simulink model "gm_ObjectTrackerHDL"  (R2024a)
settings: Solver=VariableStepAuto  StartTime=0.0  StopTime=5.5  RelTol=1e-3  EnableMultiTasking=on
PreLoadFcn:
  | % Blank input
  | img = zeros(480,640);
  | 
  | % Initialize ROI and its center
  | ROI = [175 270 127 127];
  | center = [ROI(2)+(ROI(4)+1)/2 ROI(1)+(ROI(3)+1)/2];
  | 
  | % Template Size
  | templateSize = 128;
  | tSize = templateSize;
  | 
  | % Learning rate
  | eta = 0.075;
  | 
  | % Number of training images
  | trainCount = 2;
  | 
  | % Gaussian Variance
  | sig = 2;
  | 
  | % Generate a Gaussian centered on the first frame
  | iSize = size(img);
  | [x,y] = ndgrid(1:iSize(1), 1:iSize(2));
  | gauss = exp(-((x-center(1)).^2 + (y-center(2)).^2)./(2*sig));
  | gauss = mat2gray(gauss);
  | 
  | % Generate the first template
  | img = imcrop(img, ROI);
  | gauss = imcrop(gauss, ROI);
  | 
  | % Generate the preprocess windowing function
  | [w1,w2] = meshgrid(window(@hann,tSize),window(@hann,tSize));
  | win = w1.*w2;
  | 
  | % Blank initial coefficients
  | G = zeros(tSize,tSize);
  | Ai = zeros(tSize,tSize);
  | Bi = zeros(tSize,tSize);
  | Hi = zeros(tSize,tSize);
  | 
  | numRows = tSize;
  | numCols = tSize;
InitFcn:
  | % Read the first frame
  | vidFReader = VideoReader(get_param('ObjectTrackerHDL/Input','inputFilename'));
  | img = read(vidFReader,1);
  | if (size(img,3) == 3)
  |     img = rgb2gray(img);
  | end
  | img = double(img);
  | 
  | % Initialize Object Center
  | objectCenter = str2num(get_param('ObjectTrackerHDL/ObjectTrackerHDL','objectCenter'));
  | 
  | % Template Size
  | templateSize = str2num(get_param('ObjectTrackerHDL/ObjectTrackerHDL','templateSize'));
  | originROI = objectCenter-templateSize/2;
  | tSize = templateSize;
  | 
  | % Initialize ROI and its center
  | ROI = [originROI tSize-1 tSize-1];
  | center = [ROI(2)+(ROI(4)+1)/2 ROI(1)+(ROI(3)+1)/2];
  | 
  | % Learning rate
  | eta = 0.075;
  | 
  | % Number of training images
  | trainCount = 128;
  | 
  | % Gaussian Variance
  | sig = 2;
  | 
  | % Generate a Gaussian centered on the first frame
  | iSize = size(img);
  | [x,y] = ndgrid(1:iSize(1), 1:iSize(2));
  | gauss = exp(-((x-center(1)).^2 + (y-center(2)).^2)./(2*sig));
  | gauss = mat2gray(gauss);
  | 
  | % Generate the first template
  | img = imcrop(img, ROI);
  | gauss = imcrop(gauss, ROI);
  | 
  | % Generate the preprocess windowing function
  | [w1,w2] = meshgrid(window(@hann,tSize),window(@hann,tSize));
  | win = w1.*w2;
  | 
  | % Preprocessing the first template
  | hgamma = vision.GammaCorrector(2.0,'Correction','De-gamma');
  | img = hgamma(uint8(img));
  | img = double(img);
  | mean1 = mean(img(:));
  | std1 = std(img(:));
  | img = (img-mean1)/std1;
  | fii = img.*win;
  | 
  | % Convert to frequency domain and calculate initial coefficients
  | G = fft2(gauss);
  | Ai = (G.*conj(fft2(fii)));
  | Bi = real((fft2(fii).*conj(fft2(fii))));
  | 
  | rng('default');
  | % Initial training procedure
  | for i = 1:trainCount
  | ... (+19 lines)
model workspace (MAT data in the model file):
  mwTaskManagerKernelLatency = 0
undefined symbols (not defined in the file or in its folder): a, b, c, Rec, SDTV
libraries: hdlsllib x61, simulink x17, visionhdlutilities x8, visionstatistics x6, dsphdlxfrm2 x6, visionconversions x3, visiontransforms x3, visionhdlio x2, visionhdlconversions x2, visionhdlstatistics x2, visionsinks x1, dspvision x1
(part 2 of 3)

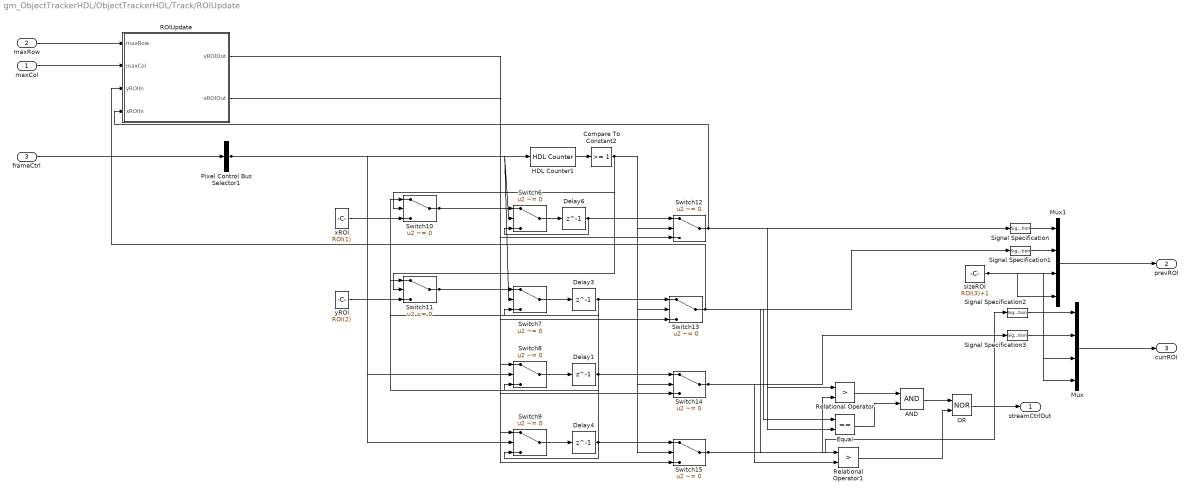
== system gm_ObjectTrackerHDL/ObjectTrackerHDL/Track/ROIUpdate ==
  maxCol : Inport  OutDataTypeStr=uint16  PortDimensions=1  SampleTime=7.94444444444444e-08
  maxRow : Inport  Port=2  OutDataTypeStr=uint16  PortDimensions=1  SampleTime=7.94444444444444e-08
  frameCtrl : Inport  Port=3
  AND : Logic  AllPortsSameDT=off  OutDataTypeStr=boolean
  Compare To Constant2 : simulink/Logic and Bit Operations/Compare To Constant  relop=>=  const=1  OutDataTypeStr=boolean
  Delay{1,3..4,6} (4 alike) : Delay  DelayLength=1
  Equal : RelationalOperator  Operator===  OutDataTypeStr=boolean  RndMeth=Simplest  InputSameDT=off
  HDL Counter1 : hdlsllib/Sources/HDL Counter  CountType=Count limited  CountInit=0  CountStep=1  CountMax=4095  CountFromType=Initial value  CountFrom=0  CountResetPort=off  CountLoadPort=off  CountEnbPort=on  CountDirPort=off  CountHitOutputPort=off  CountDataType=Unsigned  CountWordLen=12  CountFracLen=0  CountSampTime=1
  Mux : Mux
  Mux1 : Mux
  OR : Logic  Operator=NOR  AllPortsSameDT=off  OutDataTypeStr=boolean
  Pixel Control Bus Selector1 : BusSelector  OutputSignals=vEnd
  ROIUpdate : Subsystem
  Relational Operator : RelationalOperator  Operator=>  OutDataTypeStr=boolean  RndMeth=Simplest  InputSameDT=off
  Relational Operator1 : RelationalOperator  Operator=>  OutDataTypeStr=boolean  RndMeth=Simplest  InputSameDT=off
  Signal Specification{,1..3} (4 alike) : SignalSpecification  OutDataTypeStr=uint16  Dimensions=1
  Switch{6..7,10..15} (8 alike) : Switch  Criteria=u2 ~= 0  OutDataTypeStr=uint16  SaturateOnIntegerOverflow=off  InputSameDT=off
  Switch8 : Switch  Criteria=u2 ~= 0  OutDataTypeStr=fixdt(1, 17, 0)  SaturateOnIntegerOverflow=off  InputSameDT=off
  Switch9 : Switch  Criteria=u2 ~= 0  OutDataTypeStr=fixdt(1, 17, 0)  SaturateOnIntegerOverflow=off  InputSameDT=off
  sizeROI : Constant  Value=ROI(3)+1  OutDataTypeStr=uint16  SampleTime=-1
  xROI : Constant  Value=ROI(1)  OutDataTypeStr=uint16  SampleTime=-1
  yROI : Constant  Value=ROI(2)  OutDataTypeStr=uint16  SampleTime=-1
  streamCtrlOut : Outport  SampleTime=7.94444444444444e-08
  prevROI : Outport  Port=2  SampleTime=7.94444444444444e-08
  currROI : Outport  Port=3  SampleTime=7.94444444444444e-08
  wires:
  frameCtrl/1 -> Pixel Control Bus Selector1/1
  AND/1 -> OR/1
  Compare To Constant2/1 -> Switch15/2, Switch14/2, Switch13/2, Switch12/2, Switch11/2, Switch10/2
  Delay1/1 -> Switch14/1, Switch8/3, Switch11/1
  Delay4/1 -> Switch15/1, Switch9/3, Switch10/1
  Equal/1 -> AND/2
  HDL Counter1/1 -> Compare To Constant2/1
  Mux/1 -> currROI/1
  Mux1/1 -> prevROI/1
  OR/1 -> streamCtrlOut/1
  Pixel Control Bus Selector1/1 -> Switch9/2, Switch8/2, Switch7/2, Switch6/2, HDL Counter1/1
  Relational Operator/1 -> AND/1
  Relational Operator1/1 -> OR/2
  Signal Specification/1 -> Mux1/1
  Signal Specification1/1 -> Mux1/2
  Signal Specification2/1 -> Mux/1
  Signal Specification3/1 -> Mux/2
  Switch10/1 -> Switch15/3, Switch6/1, Switch12/3
  Switch11/1 -> Switch14/3, Switch7/1, Switch13/3
  Switch12/1 -> Relational Operator/1, Signal Specification/1, ROIUpdate/4(xROIIn)
  Switch13/1 -> Relational Operator1/1, Equal/1, Signal Specification1/1, ROIUpdate/3(yROIIn)
  Switch14/1 -> Relational Operator1/2, Equal/2, Signal Specification3/1
  Switch15/1 -> Relational Operator/2, Signal Specification2/1
  sizeROI/1 -> Mux1/4, Mux1/3, Mux/4, Mux/3
  Delay6/1 -> Switch12/1, Switch6/3
  Delay3/1 -> Switch13/1, Switch7/3
  xROI/1 -> Switch10/3
  yROI/1 -> Switch11/3
  maxRow/1 -> ROIUpdate/1(maxRow)
  maxCol/1 -> ROIUpdate/2(maxCol)
  Switch6/1 -> Delay6/1
  Switch8/1 -> Delay1/1
  Switch7/1 -> Delay3/1
  Switch9/1 -> Delay4/1
  ROIUpdate/1(yROIOut) -> Switch8/1
  ROIUpdate/2(xROIOut) -> Switch9/1

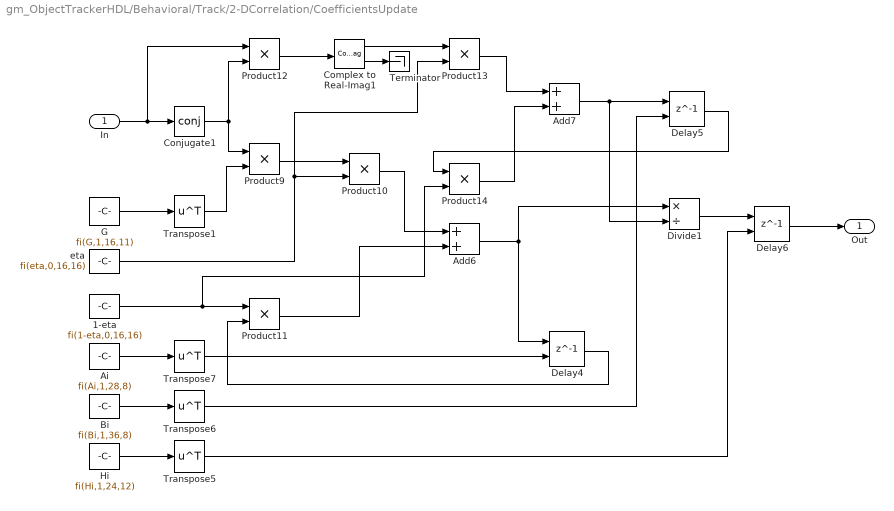
== system gm_ObjectTrackerHDL/Behavioral/Track/2-DCorrelation/CoefficientsUpdate ==
  In : Inport
  1-eta : Constant  Value=fi(1-eta,0,16,16)  OutDataTypeStr=fixdt(0,16,16)  SampleTime=-1
  Add6 : Sum  OutDataTypeStr=fixdt(1,28,8)
  Add7 : Sum  OutDataTypeStr=fixdt(1,36,8)
  Ai : Constant  Value=fi(Ai,1,28,8)  OutDataTypeStr=fixdt(1,28,8)  SampleTime=-1
  Bi : Constant  Value=fi(Bi,1,36,8)  OutDataTypeStr=fixdt(1,36,8)  SampleTime=-1
  Complex to Real-Imag1 : ComplexToRealImag
  Conjugate1 : Math  Operator=conj  SignedPower=on  RndMeth=Zero
  Delay4 : Delay  DelayLength=1  InitialConditionSource=Input port  InitialCondition=Ai
      settings: InputPortMap=u0,p4
  Delay5 : Delay  DelayLength=1  InitialConditionSource=Input port  InitialCondition=Bi
      settings: InputPortMap=u0,p4
  Delay6 : Delay  DelayLength=1  InitialConditionSource=Input port  InitialCondition=Hi
      settings: InputPortMap=u0,p4
  Divide1 : Product  Inputs=*/  OutDataTypeStr=fixdt(1,24,12)  RndMeth=Simplest  SaturateOnIntegerOverflow=on
  G : Constant  Value=fi(G,1,16,11)  VectorParams1D=off  SampleTime=-1
  Hi : Constant  Value=fi(Hi,1,24,12)  OutDataTypeStr=fixdt(1,24,12)  SampleTime=-1
  Product10 : Product  OutDataTypeStr=fixdt(1,24,12)
  Product11 : Product  OutDataTypeStr=fixdt(1,28,8)
  Product12 : Product  OutDataTypeStr=fixdt(1,32,8)
  Product13 : Product  OutDataTypeStr=fixdt(1,32,12)
  Product14 : Product  OutDataTypeStr=fixdt(1,36,8)
  Product9 : Product  OutDataTypeStr=fixdt(1,24,8)
  Terminator : Terminator
  Transpose{1,5..7} (4 alike) : Math  Operator=transpose
  eta : Constant  Value=fi(eta,0,16,16)  SampleTime=-1
  Out : Outport
  wires:
  Transpose1/1 -> Product9/2
  Delay4/1 -> Product11/2
  Transpose7/1 -> Delay4/2
  Transpose5/1 -> Delay6/2
  Product12/1 -> Complex to Real-Imag1/1
  Bi/1 -> Transpose6/1
  Delay6/1 -> Out/1
  Complex to Real-Imag1/1 -> Product13/1
  Complex to Real-Imag1/2 -> Terminator/1
  G/1 -> Transpose1/1
  Product13/1 -> Add7/1
  Delay5/1 -> Product14/1
  Product10/1 -> Add6/1
  Hi/1 -> Transpose5/1
  Add7/1 -> Divide1/2, Delay5/1
  Transpose6/1 -> Delay5/2
  1-eta/1 -> Product14/2, Product11/1
  Product11/1 -> Add6/2
  Conjugate1/1 -> Product9/1, Product12/2
  Product9/1 -> Product10/1
  In/1 -> Conjugate1/1, Product12/1
  eta/1 -> Product10/2, Product13/2
  Divide1/1 -> Delay6/1
  Add6/1 -> Divide1/1, Delay4/1
  Ai/1 -> Transpose7/1
  Product14/1 -> Add7/2

== system gm_ObjectTrackerHDL/Behavioral/Track/ROIUpdate/CurrValidROI ==
  ROIIn : Inport
  Constant : Constant  Value=iSize(1)-tSize  OutDataTypeStr=uint16  SampleTime=-1
  Constant1 : Constant  Value=iSize(2)-tSize  OutDataTypeStr=uint16  SampleTime=-1
  Demux : Demux
  Mux1 : Mux
  Relational Operator : RelationalOperator  Operator=<  OutDataTypeStr=boolean  RndMeth=Simplest  InputSameDT=off
  Relational Operator1 : RelationalOperator  Operator=<  OutDataTypeStr=boolean  RndMeth=Simplest  InputSameDT=off
  Switch : Switch  Criteria=u2 ~= 0  SaturateOnIntegerOverflow=off  InputSameDT=off
  Switch1 : Switch  Criteria=u2 ~= 0  SaturateOnIntegerOverflow=off  InputSameDT=off
  ROIOut : Outport
  wires:
  Switch1/1 -> Mux1/2
  Relational Operator1/1 -> Switch1/2
  Switch/1 -> Mux1/1
  Relational Operator/1 -> Switch/2
  Demux/4 -> Mux1/4
  Demux/3 -> Mux1/3
  Constant/1 -> Relational Operator1/2, Switch1/3
  Demux/2 -> Switch1/1, Relational Operator1/1
  Constant1/1 -> Relational Operator/2, Switch/3
  Demux/1 -> Relational Operator/1, Switch/1
  ROIIn/1 -> Demux/1
  Mux1/1 -> ROIOut/1

== system gm_ObjectTrackerHDL/Behavioral/Track/ROIUpdate/PrevValidROI ==
  ROIIn : Inport
  Constant : Constant  Value=iSize(1)-tSize  OutDataTypeStr=uint16  SampleTime=-1
  Constant1 : Constant  Value=iSize(2)-tSize  OutDataTypeStr=uint16  SampleTime=-1
  Demux : Demux
  Mux1 : Mux
  Relational Operator : RelationalOperator  Operator=<  OutDataTypeStr=boolean  RndMeth=Simplest  InputSameDT=off
  Relational Operator1 : RelationalOperator  Operator=<  OutDataTypeStr=boolean  RndMeth=Simplest  InputSameDT=off
  Switch : Switch  Criteria=u2 ~= 0  SaturateOnIntegerOverflow=off  InputSameDT=off
  Switch1 : Switch  Criteria=u2 ~= 0  SaturateOnIntegerOverflow=off  InputSameDT=off
  ROIOut : Outport
  wires:
  Switch1/1 -> Mux1/2
  Relational Operator1/1 -> Switch1/2
  Switch/1 -> Mux1/1
  Relational Operator/1 -> Switch/2
  Demux/4 -> Mux1/4
  Demux/3 -> Mux1/3
  Constant/1 -> Relational Operator1/2, Switch1/3
  Demux/2 -> Switch1/1, Relational Operator1/1
  Constant1/1 -> Relational Operator/2, Switch/3
  Demux/1 -> Relational Operator/1, Switch/1
  ROIIn/1 -> Demux/1
  Mux1/1 -> ROIOut/1

== system gm_ObjectTrackerHDL/ObjectTrackerHDL/Overlay/VideoOverlay/Divide ==
  In1 : Inport
  In2 : Inport  Port=2
  Divide : Product  Inputs=*/  OutDataTypeStr=fixdt(1, 18, 0)  RndMeth=Zero  SaturateOnIntegerOverflow=on
  Divide_pd1 : Delay  DelayLength=22
  Out1 : Outport
  wires:
  In1/1 -> Divide/1
  In2/1 -> Divide/2
  Divide/1 -> Divide_pd1/1
  Divide_pd1/1 -> Out1/1

== system gm_ObjectTrackerHDL/ObjectTrackerHDL/Overlay/VideoOverlay/MATLAB Function ==
  position : Inport  OutDataTypeStr=uint16  PortDimensions=[1 4]  SampleTime=7.94444444444444e-08
  rowCount : Inport  Port=2  OutDataTypeStr=int32  PortDimensions=1  SampleTime=7.94444444444444e-08
  colCount : Inport  Port=3  OutDataTypeStr=int32  PortDimensions=1  SampleTime=7.94444444444444e-08
  colorValue : Inport  Port=4  OutDataTypeStr=uint8  PortDimensions=[1 3]  SampleTime=7.94444444444444e-08
  lineWidth : Inport  Port=5  OutDataTypeStr=uint8  PortDimensions=1  SampleTime=7.94444444444444e-08
  MATLAB Function : MATLAB Function  TreatAsAtomicUnit=on
  Color : Outport  SampleTime=7.94444444444444e-08  VectorParamsAs1DForOutWhenUnconnected=off
  AddShape : Outport  Port=2  SampleTime=7.94444444444444e-08
  wires:
  position/1 -> MATLAB Function/1(position)
  rowCount/1 -> MATLAB Function/2(rowCount)
  colCount/1 -> MATLAB Function/3(colCount)
  colorValue/1 -> MATLAB Function/4(colorValue)
  lineWidth/1 -> MATLAB Function/5(lineWidth)
  MATLAB Function/1(Color) -> Color/1
  MATLAB Function/2(AddShape) -> AddShape/1

== system gm_ObjectTrackerHDL/ObjectTrackerHDL/Preprocess/CurrPreprocess/Divide1 ==
  In1 : Inport
  In2 : Inport  Port=2
  Divide1 : Product  Inputs=*/  OutDataTypeStr=fixdt(1,16,12)  RndMeth=Zero  SaturateOnIntegerOverflow=on
  Divide1_pd1 : Delay  DelayLength=34
  Out1 : Outport
  wires:
  In1/1 -> Divide1/1
  In2/1 -> Divide1/2
  Divide1/1 -> Divide1_pd1/1
  Divide1_pd1/1 -> Out1/1

== system gm_ObjectTrackerHDL/ObjectTrackerHDL/Preprocess/CurrPreprocess/Multiply_ShiftAdd_inst ==
  In1 : Inport
  In2 : Inport  Port=2
  Multiply_ShiftAdd_inst : Product  OutDataTypeStr=fixdt(1, 32, 28)
  Multiply_ShiftAdd_inst_pd1 : Delay  DelayLength=4
  Out1 : Outport
  wires:
  In1/1 -> Multiply_ShiftAdd_inst/1
  In2/1 -> Multiply_ShiftAdd_inst/2
  Multiply_ShiftAdd_inst_pd1/1 -> Out1/1
  Multiply_ShiftAdd_inst/1 -> Multiply_ShiftAdd_inst_pd1/1

== system gm_ObjectTrackerHDL/ObjectTrackerHDL/Preprocess/PrevPreprocess/Divide2 ==
  In1 : Inport
  In2 : Inport  Port=2
  Divide2 : Product  Inputs=*/  OutDataTypeStr=fixdt(1,16,12)  RndMeth=Zero  SaturateOnIntegerOverflow=on
  Divide2_pd1 : Delay  DelayLength=34
  Out1 : Outport
  wires:
  In1/1 -> Divide2/1
  In2/1 -> Divide2/2
  Divide2/1 -> Divide2_pd1/1
  Divide2_pd1/1 -> Out1/1

== system gm_ObjectTrackerHDL/ObjectTrackerHDL/Preprocess/PrevPreprocess/Multiply_ShiftAdd_inst ==
  In1 : Inport
  In2 : Inport  Port=2
  Multiply_ShiftAdd_inst : Product  OutDataTypeStr=fixdt(1, 32, 28)
  Multiply_ShiftAdd_inst_pd1 : Delay  DelayLength=4
  Out1 : Outport
  wires:
  In1/1 -> Multiply_ShiftAdd_inst/1
  In2/1 -> Multiply_ShiftAdd_inst/2
  Multiply_ShiftAdd_inst_pd1/1 -> Out1/1
  Multiply_ShiftAdd_inst/1 -> Multiply_ShiftAdd_inst_pd1/1

== system gm_ObjectTrackerHDL/ObjectTrackerHDL/Track/2-DCorrelation/2-DIFFT ==
  pixelIn : Inport  OutDataTypeStr=fixdt(1, 24, 16)  PortDimensions=1  SampleTime=7.94444444444444e-08
      settings: SignalType=complex
  ctrlIn : Inport  Port=2
  " " : DataTypeConversion  OutDataTypeStr=fixdt(1,24,16)  SaturateOnIntegerOverflow=off  RndMeth=Floor
  Bit Concat1 : hdlsllib/Logic and Bit Operations/Bit Concat  numInputs=2
  Bit Slice4 : hdlsllib/Logic and Bit Operations/Bit Slice  lidx=31  ridx=0
  Bit Slice5 : hdlsllib/Logic and Bit Operations/Bit Slice  lidx=63  ridx=32
  ColumnIFFT : dsphdlxfrm2/IFFT  Architecture=Streaming Radix 2^2  FFTLengthSource=Property  FFTLength=tSize  FFTLengthMax=1024  ComplexMultiplication=Use 4 multipliers and 2 adders  BitReversedOutput=off  BitReversedInput=off  Normalize=on  SimulateUsing=Code generation  RoundingMethod=Floor  ResetInputPort=off  StartOutputPort=off  EndOutputPort=off
  Complex to Real-Imag : ComplexToRealImag
  Complex to Real-Imag1 : ComplexToRealImag
  Complex to Real-Imag_term1 : Terminator
  CornerTurnMemory : Subsystem
  Data Type Conversion10 : DataTypeConversion  OutDataTypeStr=fixdt(1,24,16)  SaturateOnIntegerOverflow=off  RndMeth=Floor
  Data Type Conversion12 : DataTypeConversion  OutDataTypeStr=fixdt(1,24,16)  SaturateOnIntegerOverflow=off  RndMeth=Floor
  Data Type Conversion8 : DataTypeConversion  OutDataTypeStr=fixdt(0,32,0)  ConvertRealWorld=Stored Integer (SI)  SaturateOnIntegerOverflow=off  RndMeth=Floor
  Data Type Conversion9 : DataTypeConversion  OutDataTypeStr=fixdt(1,24,16)  ConvertRealWorld=Stored Integer (SI)  SaturateOnIntegerOverflow=off  RndMeth=Floor
  Pixel Control Bus Selector1 : BusSelector  OutputSignals=valid
  Real-Imag to Complex1 : RealImagToComplex
  RowIFFT : dsphdlxfrm2/IFFT  Architecture=Streaming Radix 2^2  FFTLengthSource=Property  FFTLength=tSize  FFTLengthMax=1024  ComplexMultiplication=Use 4 multipliers and 2 adders  BitReversedOutput=off  BitReversedInput=off  Normalize=on  SimulateUsing=Code generation  RoundingMethod=Floor  ResetInputPort=off  StartOutputPort=off  EndOutputPort=off
  pixelBusGenerator : Subsystem  mask{hEnd=double(127), vEnd=double(16383)}
      mask prompts: hEnd "hEnd Count"; vEnd "vEnd Count"
  pixelOut : Outport  SampleTime=7.94444444444444e-08
  ctrlOut : Outport  Port=2
  wires:
  pixelIn/1 -> Data Type Conversion10/1
  ctrlIn/1 -> Pixel Control Bus Selector1/1
  " "/1 -> Complex to Real-Imag/1
  Bit Concat1/1 -> CornerTurnMemory/1(dataIn)
  Bit Slice4/1 -> Real-Imag to Complex1/2
  Bit Slice5/1 -> Real-Imag to Complex1/1
  ColumnIFFT/1 -> " "/1
  ColumnIFFT/2 -> pixelBusGenerator/1(validIn)
  Complex to Real-Imag/1 -> pixelOut/1
  Complex to Real-Imag/2 -> Complex to Real-Imag_term1/1
  Complex to Real-Imag1/1 -> Bit Concat1/1
  Complex to Real-Imag1/2 -> Bit Concat1/2
  CornerTurnMemory/1(dataOut) -> Bit Slice5/1, Bit Slice4/1
  CornerTurnMemory/2(validOut) -> ColumnIFFT/2
  Data Type Conversion10/1 -> RowIFFT/1
  Data Type Conversion12/1 -> Data Type Conversion8/1
  Data Type Conversion8/1 -> Complex to Real-Imag1/1
  Data Type Conversion9/1 -> ColumnIFFT/1
  Pixel Control Bus Selector1/1 -> RowIFFT/2
  Real-Imag to Complex1/1 -> Data Type Conversion9/1
  RowIFFT/1 -> Data Type Conversion12/1
  RowIFFT/2 -> CornerTurnMemory/2(validIn)
  pixelBusGenerator/1(busOut) -> ctrlOut/1

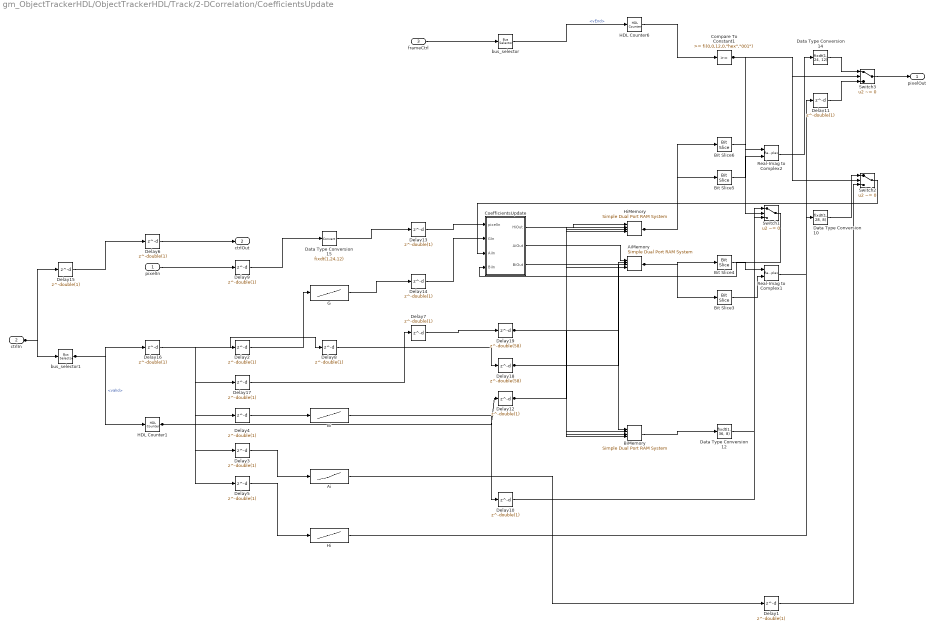
== system gm_ObjectTrackerHDL/ObjectTrackerHDL/Track/2-DCorrelation/CoefficientsUpdate ==
  pixelIn : Inport  OutDataTypeStr=fixdt(1, 24, 12)  PortDimensions=1  SampleTime=7.94444444444444e-08
      settings: SignalType=complex
  ctrlIn : Inport  Port=2
  frameCtrl : Inport  Port=3
  Ai : Lookup_n-D  NumberOfTableDimensions=1  LookupTableObject=''  BreakpointsForDimension1=[0:tSize * tSize - 1]  BreakpointsForDimension1FirstPoint=10  BreakpointsForDimension2FirstPoint=10  BreakpointsForDimension1Spacing=12  BreakpointsForDimension2Spacing=12  IndexSearchMethod=Evenly spaced points  Table=fi(Ai(:),1,28,8)  InterpMethod=Flat  InternalRulePriority=Speed  OutDataTypeStr=fixdt(1,28,8)  RndMeth=Simplest
  AiMemory : hdlsllib/HDL RAMs/Simple Dual Port RAM System  RAMType=Simple dual port  AsyncRead=off  WriteOutputValue=New data  RAMInitialValue=0  allowBusInputs=off  WritesHaveOutput=on  NumReads=0  NumWrites=1  SimulateUsing=Code generation
  Bi : Lookup_n-D  NumberOfTableDimensions=1  LookupTableObject=''  BreakpointsForDimension1=[0:tSize * tSize - 1]  BreakpointsForDimension1FirstPoint=10  BreakpointsForDimension2FirstPoint=10  BreakpointsForDimension1Spacing=12  BreakpointsForDimension2Spacing=12  IndexSearchMethod=Evenly spaced points  Table=fi(Bi(:),1,36,8)  InterpMethod=Flat  InternalRulePriority=Speed  OutDataTypeStr=fixdt(1,36,8)  RndMeth=Simplest
  BiMemory : hdlsllib/HDL RAMs/Simple Dual Port RAM System  RAMType=Simple dual port  AsyncRead=off  WriteOutputValue=New data  RAMInitialValue=0  allowBusInputs=off  WritesHaveOutput=on  NumReads=0  NumWrites=1  SimulateUsing=Code generation
  Bit Slice3 : hdlsllib/Logic and Bit Operations/Bit Slice  lidx=double(31)  ridx=double(0)
  Bit Slice4 : hdlsllib/Logic and Bit Operations/Bit Slice  lidx=double(63)  ridx=double(32)
  Bit Slice5 : hdlsllib/Logic and Bit Operations/Bit Slice  lidx=double(31)  ridx=double(0)
  Bit Slice6 : hdlsllib/Logic and Bit Operations/Bit Slice  lidx=double(63)  ridx=double(32)
  CoefficientsUpdate : Subsystem
  Compare To Constant1 : simulink/Logic and Bit Operations/Compare To Constant  relop=>=  const="fi(0,0,12,0,\"hex\",\"001\")"  OutDataTypeStr=boolean
  Data Type Conversion10 : DataTypeConversion  OutDataTypeStr=fixdt(1, 28, 8)  ConvertRealWorld=Stored Integer (SI)  SampleTime=7.94444444444444e-08  SaturateOnIntegerOverflow=off  RndMeth=Floor
  Data Type Conversion12 : DataTypeConversion  OutDataTypeStr=fixdt(1, 36, 8)  ConvertRealWorld=Stored Integer (SI)  SampleTime=7.94444444444444e-08  SaturateOnIntegerOverflow=off  RndMeth=Floor
  Data Type Conversion14 : DataTypeConversion  OutDataTypeStr=fixdt(1, 24, 12)  ConvertRealWorld=Stored Integer (SI)  SampleTime=7.94444444444444e-08  SaturateOnIntegerOverflow=off  RndMeth=Floor
  Data Type Conversion15 : DataTypeConversion  OutDataTypeStr=fixdt(1,24,12)
  Delay{1..5,7..14,16..17} (15 alike) : Delay  DelayLength=double(1)  InitialCondition=0  SampleTime=7.94444444444444e-08
  Delay15 : Delay  DelayLength=double(1)  SampleTime=7.94444444444444e-08
  Delay18 : Delay  DelayLength=double(58)  InitialCondition=0  SampleTime=7.94444444444444e-08
  Delay19 : Delay  DelayLength=double(58)  InitialCondition=0  SampleTime=7.94444444444444e-08
  Delay6 : Delay  DelayLength=double(1)  SampleTime=7.94444444444444e-08
  G : Lookup_n-D  NumberOfTableDimensions=1  LookupTableObject=''  BreakpointsForDimension1=[0:tSize * tSize - 1]  BreakpointsForDimension1FirstPoint=10  BreakpointsForDimension2FirstPoint=10  BreakpointsForDimension1Spacing=12  BreakpointsForDimension2Spacing=12  IndexSearchMethod=Evenly spaced points  Table=fi(G(:),1,16,11)  InterpMethod=Flat  InternalRulePriority=Speed  OutDataTypeStr=fixdt(1,16,11)  RndMeth=Simplest
  HDL Counter1 : hdlsllib/Sources/HDL Counter  CountType=Count limited  CountInit=0  CountStep=1  CountMax=tSize * tSize - 1  CountFromType=Initial value  CountFrom=0  CountResetPort=off  CountLoadPort=off  CountEnbPort=on  CountDirPort=off  CountHitOutputPort=off  CountDataType=Unsigned  CountWordLen=ceil(log2(tSize * tSize - 1))  CountFracLen=0  CountSampTime=1
  HDL Counter6 : hdlsllib/Sources/HDL Counter  CountType=Count limited  CountInit=0  CountStep=1  CountMax=4095  CountFromType=Initial value  CountFrom=0  CountResetPort=off  CountLoadPort=off  CountEnbPort=on  CountDirPort=off  CountHitOutputPort=off  CountDataType=Unsigned  CountWordLen=12  CountFracLen=0  CountSampTime=1
  Hi : Lookup_n-D  NumberOfTableDimensions=1  LookupTableObject=''  BreakpointsForDimension1=[0:tSize * tSize - 1]  BreakpointsForDimension1FirstPoint=10  BreakpointsForDimension2FirstPoint=10  BreakpointsForDimension1Spacing=12  BreakpointsForDimension2Spacing=12  IndexSearchMethod=Evenly spaced points  Table=fi(Hi(:),1,24,12)  InterpMethod=Flat  InternalRulePriority=Speed  OutDataTypeStr=fixdt(1,24,12)  RndMeth=Simplest
  HiMemory : hdlsllib/HDL RAMs/Simple Dual Port RAM System  RAMType=Simple dual port  AsyncRead=off  WriteOutputValue=New data  RAMInitialValue=0  allowBusInputs=off  WritesHaveOutput=on  NumReads=0  NumWrites=1  SimulateUsing=Code generation
  Real-Imag to Complex1 : RealImagToComplex  ConstantPart="fi(0,0,32,0,\"hex\",\"00000000\")"  SampleTime=7.94444444444444e-08
  Real-Imag to Complex2 : RealImagToComplex  ConstantPart="fi(0,0,32,0,\"hex\",\"00000000\")"  SampleTime=7.94444444444444e-08
  Switch1 : Switch  Criteria=u2 ~= 0  Threshold=double(0)  OutDataTypeStr=fixdt(1, 36, 8)  SampleTime=7.94444444444444e-08  SaturateOnIntegerOverflow=off  InputSameDT=off
  Switch2 : Switch  Criteria=u2 ~= 0  Threshold=double(0)  OutDataTypeStr=fixdt(1, 28, 8)  SampleTime=7.94444444444444e-08  SaturateOnIntegerOverflow=off  InputSameDT=off
  Switch3 : Switch  Criteria=u2 ~= 0  Threshold=double(0)  OutDataTypeStr=fixdt(1, 24, 12)  SampleTime=7.94444444444444e-08  SaturateOnIntegerOverflow=off  InputSameDT=off
  bus_selector : BusSelector  OutputSignals=vEnd
  bus_selector1 : BusSelector  OutputSignals=valid
  pixelOut : Outport  SampleTime=7.94444444444444e-08
  ctrlOut : Outport  Port=2
  wires:
  pixelIn/1 -> Delay9/1
  ctrlIn/1 -> bus_selector1/1, Delay15/1
  frameCtrl/1 -> bus_selector/1
  Ai/1 -> Delay1/1
  Bi/1 -> Delay10/1
  Bit Slice5/1 -> Real-Imag to Complex2/2
  Bit Slice6/1 -> Real-Imag to Complex2/1
  CoefficientsUpdate/1(HiOut) -> HiMemory/1
  Compare To Constant1/1 -> Switch3/2, Switch1/2, Switch2/2
  Data Type Conversion14/1 -> Switch3/1
  Data Type Conversion15/1 -> Delay13/1
  Delay11/1 -> Switch3/3
  Delay12/1 -> AiMemory/4, HiMemory/4, BiMemory/4
  Delay15/1 -> Delay6/1
  Delay16/1 -> Delay8/1
  Delay17/1 -> Delay7/1
  Delay18/1 -> AiMemory/3, HiMemory/3, BiMemory/3
  Delay19/1 -> AiMemory/2, HiMemory/2, BiMemory/2
  Delay2/1 -> G/1
  Delay3/1 -> Ai/1
  Delay4/1 -> Bi/1
  Delay5/1 -> Hi/1
  Delay6/1 -> ctrlOut/1
  Delay7/1 -> Delay19/1
  Delay8/1 -> Delay18/1
  Delay9/1 -> Data Type Conversion15/1
  G/1 -> Delay14/1
  HDL Counter1/1 -> Delay5/1, Delay4/1, Delay3/1, Delay2/1, Delay17/1, Delay12/1
  HDL Counter6/1 -> Compare To Constant1/1
  Hi/1 -> Delay11/1
  HiMemory/1 -> Bit Slice6/1, Bit Slice5/1
  bus_selector/1 -> HDL Counter6/1  "<vEnd>"
  bus_selector1/1 -> Delay16/1, HDL Counter1/1  "<valid>"
  Real-Imag to Complex2/1 -> Data Type Conversion14/1
  Switch3/1 -> pixelOut/1
  CoefficientsUpdate/2(AiOut) -> AiMemory/1
  AiMemory/1 -> Bit Slice4/1, Bit Slice3/1
  Bit Slice4/1 -> Real-Imag to Complex1/1
  Real-Imag to Complex1/1 -> Data Type Conversion10/1
  Data Type Conversion10/1 -> Switch2/1
  CoefficientsUpdate/3(BiOut) -> BiMemory/1
  Delay13/1 -> CoefficientsUpdate/1(pixelIn)
  Delay14/1 -> CoefficientsUpdate/2(GIn)
  Delay10/1 -> Switch1/3
  Bit Slice3/1 -> Real-Imag to Complex1/2
  Switch2/1 -> CoefficientsUpdate/3(AiIn)
  Delay1/1 -> Switch2/3
  Switch1/1 -> CoefficientsUpdate/4(BiIn)
  BiMemory/1 -> Data Type Conversion12/1
  Data Type Conversion12/1 -> Switch1/1

== system gm_ObjectTrackerHDL/ObjectTrackerHDL/Track/2-DCorrelation/Curr2-DFFT ==
  pixelIn : Inport  OutDataTypeStr=fixdt(1, 32, 28)  PortDimensions=1  SampleTime=7.94444444444444e-08
  ctrlIn : Inport  Port=2
  " " : DataTypeConversion  OutDataTypeStr=fixdt(1,24,12)  SaturateOnIntegerOverflow=off  RndMeth=Floor
  Bit Concat : hdlsllib/Logic and Bit Operations/Bit Concat  numInputs=2
  Bit Slice1 : hdlsllib/Logic and Bit Operations/Bit Slice  lidx=31  ridx=0
  Bit Slice2 : hdlsllib/Logic and Bit Operations/Bit Slice  lidx=63  ridx=32
  ColumnFFT : dsphdlxfrm2/FFT  Architecture=Streaming Radix 2^2  FFTLengthSource=Property  FFTLength=tSize  FFTLengthMax=1024  ComplexMultiplication=Use 4 multipliers and 2 adders  BitReversedOutput=off  BitReversedInput=off  Normalize=off  SimulateUsing=Code generation  RoundingMethod=Floor  ResetInputPort=off  StartOutputPort=off  EndOutputPort=off
  Complex to Real-Imag1 : ComplexToRealImag
  CornerTurnMemory : Subsystem
  Data Type Conversion2 : DataTypeConversion  OutDataTypeStr=fixdt(0,32,0)  ConvertRealWorld=Stored Integer (SI)  SaturateOnIntegerOverflow=off  RndMeth=Floor
  Data Type Conversion3 : DataTypeConversion  OutDataTypeStr=fixdt(1,28,16)  ConvertRealWorld=Stored Integer (SI)  SaturateOnIntegerOverflow=off  RndMeth=Floor
  Data Type Conversion6 : DataTypeConversion  OutDataTypeStr=fixdt(1,28,16)  SaturateOnIntegerOverflow=off  RndMeth=Floor
  Pixel Control Bus Selector1 : BusSelector  OutputSignals=valid
  Real-Imag to Complex : RealImagToComplex
  RowFFT : dsphdlxfrm2/FFT  Architecture=Streaming Radix 2^2  FFTLengthSource=Property  FFTLength=tSize  FFTLengthMax=1024  ComplexMultiplication=Use 4 multipliers and 2 adders  BitReversedOutput=off  BitReversedInput=off  Normalize=off  SimulateUsing=Code generation  RoundingMethod=Floor  ResetInputPort=off  StartOutputPort=off  EndOutputPort=off
  pixelBusGenerator : Subsystem  mask{hEnd=double(127), vEnd=double(16383)}
      mask prompts: hEnd "hEnd Count"; vEnd "vEnd Count"
  pixelOut : Outport  SampleTime=7.94444444444444e-08
  ctrlOut : Outport  Port=2
  wires:
  pixelIn/1 -> RowFFT/1
  ctrlIn/1 -> Pixel Control Bus Selector1/1
  " "/1 -> pixelOut/1
  Bit Concat/1 -> CornerTurnMemory/1(dataIn)
  Bit Slice1/1 -> Real-Imag to Complex/2
  Bit Slice2/1 -> Real-Imag to Complex/1
  ColumnFFT/1 -> " "/1
  ColumnFFT/2 -> pixelBusGenerator/1(validIn)
  Complex to Real-Imag1/1 -> Bit Concat/1
  Complex to Real-Imag1/2 -> Bit Concat/2
  CornerTurnMemory/1(dataOut) -> Bit Slice2/1, Bit Slice1/1
  CornerTurnMemory/2(validOut) -> ColumnFFT/2
  Data Type Conversion2/1 -> Complex to Real-Imag1/1
  Data Type Conversion3/1 -> ColumnFFT/1
  Data Type Conversion6/1 -> Data Type Conversion2/1
  Pixel Control Bus Selector1/1 -> RowFFT/2
  Real-Imag to Complex/1 -> Data Type Conversion3/1
  RowFFT/1 -> Data Type Conversion6/1
  RowFFT/2 -> CornerTurnMemory/2(validIn)
  pixelBusGenerator/1(busOut) -> ctrlOut/1

== system gm_ObjectTrackerHDL/ObjectTrackerHDL/Track/2-DCorrelation/Prev2-DFFT ==
  pixelIn : Inport  OutDataTypeStr=fixdt(1, 32, 28)  PortDimensions=1  SampleTime=7.94444444444444e-08
  ctrlIn : Inport  Port=2
  " " : DataTypeConversion  OutDataTypeStr=fixdt(1,24,12)  SaturateOnIntegerOverflow=off  RndMeth=Floor
  Bit Concat : hdlsllib/Logic and Bit Operations/Bit Concat  numInputs=2
  Bit Slice1 : hdlsllib/Logic and Bit Operations/Bit Slice  lidx=31  ridx=0
  Bit Slice2 : hdlsllib/Logic and Bit Operations/Bit Slice  lidx=63  ridx=32
  ColumnFFT : dsphdlxfrm2/FFT  Architecture=Streaming Radix 2^2  FFTLengthSource=Property  FFTLength=tSize  FFTLengthMax=1024  ComplexMultiplication=Use 4 multipliers and 2 adders  BitReversedOutput=off  BitReversedInput=off  Normalize=off  SimulateUsing=Code generation  RoundingMethod=Floor  ResetInputPort=off  StartOutputPort=off  EndOutputPort=off
  Complex to Real-Imag1 : ComplexToRealImag
  CornerTurnMemory : Subsystem
  Data Type Conversion2 : DataTypeConversion  OutDataTypeStr=fixdt(0,32,0)  ConvertRealWorld=Stored Integer (SI)  SaturateOnIntegerOverflow=off  RndMeth=Floor
  Data Type Conversion3 : DataTypeConversion  OutDataTypeStr=fixdt(1,28,16)  ConvertRealWorld=Stored Integer (SI)  SaturateOnIntegerOverflow=off  RndMeth=Floor
  Data Type Conversion6 : DataTypeConversion  OutDataTypeStr=fixdt(1,28,16)  SaturateOnIntegerOverflow=off  RndMeth=Floor
  Pixel Control Bus Selector1 : BusSelector  OutputSignals=valid
  Real-Imag to Complex : RealImagToComplex
  RowFFT : dsphdlxfrm2/FFT  Architecture=Streaming Radix 2^2  FFTLengthSource=Property  FFTLength=tSize  FFTLengthMax=1024  ComplexMultiplication=Use 4 multipliers and 2 adders  BitReversedOutput=off  BitReversedInput=off  Normalize=off  SimulateUsing=Code generation  RoundingMethod=Floor  ResetInputPort=off  StartOutputPort=off  EndOutputPort=off
  pixelBusGenerator : Subsystem  mask{hEnd=double(127), vEnd=double(16383)}
      mask prompts: hEnd "hEnd Count"; vEnd "vEnd Count"
  pixelOut : Outport  SampleTime=7.94444444444444e-08
  ctrlOut : Outport  Port=2
  wires:
  pixelIn/1 -> RowFFT/1
  ctrlIn/1 -> Pixel Control Bus Selector1/1
  " "/1 -> pixelOut/1
  Bit Concat/1 -> CornerTurnMemory/1(dataIn)
  Bit Slice1/1 -> Real-Imag to Complex/2
  Bit Slice2/1 -> Real-Imag to Complex/1
  ColumnFFT/1 -> " "/1
  ColumnFFT/2 -> pixelBusGenerator/1(validIn)
  Complex to Real-Imag1/1 -> Bit Concat/1
  Complex to Real-Imag1/2 -> Bit Concat/2
  CornerTurnMemory/1(dataOut) -> Bit Slice2/1, Bit Slice1/1
  CornerTurnMemory/2(validOut) -> ColumnFFT/2
  Data Type Conversion2/1 -> Complex to Real-Imag1/1
  Data Type Conversion3/1 -> ColumnFFT/1
  Data Type Conversion6/1 -> Data Type Conversion2/1
  Pixel Control Bus Selector1/1 -> RowFFT/2
  Real-Imag to Complex/1 -> Data Type Conversion3/1
  RowFFT/1 -> Data Type Conversion6/1
  RowFFT/2 -> CornerTurnMemory/2(validIn)
  pixelBusGenerator/1(busOut) -> ctrlOut/1

== system gm_ObjectTrackerHDL/ObjectTrackerHDL/Track/2-DCorrelation/StreamAlignment ==
  pixelIn1 : Inport  OutDataTypeStr=fixdt(1, 24, 12)  PortDimensions=1  SampleTime=7.94444444444444e-08
      settings: SignalType=complex
  ctrlIn1 : Inport  Port=2
  pixelIn2 : Inport  Port=3  OutDataTypeStr=fixdt(1, 24, 12)  PortDimensions=1  SampleTime=7.94444444444444e-08
      settings: SignalType=complex
  ctrlIn2 : Inport  Port=4
  streamCtrl : Inport  Port=5  OutDataTypeStr=boolean  PortDimensions=1  SampleTime=7.94444444444444e-08
  Complex to Real-Imag : ComplexToRealImag
  Complex to Real-Imag1 : ComplexToRealImag
  Pixel Stream Aligner : visionhdlutilities/Pixel Stream Aligner  LineBufferSize=256  MaximumNumberOfLines=tSize  SimulateUsing=Code generation
  Pixel Stream Aligner1 : visionhdlutilities/Pixel Stream Aligner  LineBufferSize=256  MaximumNumberOfLines=tSize  SimulateUsing=Code generation
  Pixel Stream Aligner1_term2 : Terminator
  Real-Imag to Complex : RealImagToComplex
  Real-Imag to Complex1 : RealImagToComplex
  Switch2 : Switch  Criteria=u2 ~= 0  OutDataTypeStr=fixdt(1, 24, 12)  SaturateOnIntegerOverflow=off  InputSameDT=off
  Switch3 : Switch  Criteria=u2 ~= 0  SaturateOnIntegerOverflow=off  InputSameDT=off
  Switch4 : Switch  Criteria=u2 ~= 0  OutDataTypeStr=fixdt(1, 24, 12)  SaturateOnIntegerOverflow=off  InputSameDT=off
  Switch5 : Switch  Criteria=u2 ~= 0  SaturateOnIntegerOverflow=off  InputSameDT=off
  pixelOut1 : Outport  SampleTime=7.94444444444444e-08
  pixelOut2 : Outport  Port=2  SampleTime=7.94444444444444e-08
  ctrlOut : Outport  Port=3
  wires:
  pixelIn1/1 -> Switch4/3, Switch2/1
  ctrlIn1/1 -> Switch5/3, Switch3/1
  pixelIn2/1 -> Switch4/1, Switch2/3
  ctrlIn2/1 -> Switch5/1, Switch3/3
  streamCtrl/1 -> Switch5/2, Switch4/2, Switch3/2, Switch2/2
  Complex to Real-Imag/1 -> Pixel Stream Aligner/1
  Complex to Real-Imag/2 -> Pixel Stream Aligner1/1
  Complex to Real-Imag1/1 -> Pixel Stream Aligner/3
  Complex to Real-Imag1/2 -> Pixel Stream Aligner1/3
  Pixel Stream Aligner/1 -> Real-Imag to Complex/1
  Pixel Stream Aligner/2 -> Real-Imag to Complex1/1
  Pixel Stream Aligner/3 -> ctrlOut/1
  Pixel Stream Aligner1/1 -> Real-Imag to Complex/2
  Pixel Stream Aligner1/2 -> Real-Imag to Complex1/2
  Pixel Stream Aligner1/3 -> Pixel Stream Aligner1_term2/1
  Real-Imag to Complex/1 -> pixelOut1/1
  Real-Imag to Complex1/1 -> pixelOut2/1
  Switch2/1 -> Complex to Real-Imag/1
  Switch3/1 -> Pixel Stream Aligner/2, Pixel Stream Aligner1/2
  Switch4/1 -> Complex to Real-Imag1/1
  Switch5/1 -> Pixel Stream Aligner/4, Pixel Stream Aligner1/4

== system gm_ObjectTrackerHDL/ObjectTrackerHDL/Track/MaxCorrelation/Divide2 ==
  In1 : Inport
  In2 : Inport  Port=2
  Divide2 : Product  Inputs=*/  OutDataTypeStr=uint16  RndMeth=Zero  SaturateOnIntegerOverflow=on
  Divide2_pd1 : Delay  DelayLength=20
  Out1 : Outport
  wires:
  In2/1 -> Divide2/2
  In1/1 -> Divide2/1
  Divide2/1 -> Divide2_pd1/1
  Divide2_pd1/1 -> Out1/1

== system gm_ObjectTrackerHDL/ObjectTrackerHDL/Track/MaxCorrelation/Divide3 ==
  In1 : Inport
  In2 : Inport  Port=2
  Divide3 : Product  Inputs=*/  OutDataTypeStr=uint16  RndMeth=Zero  SaturateOnIntegerOverflow=on
  Divide3_pd1 : Delay  DelayLength=20
  Out1 : Outport
  wires:
  In1/1 -> Divide3/1
  In2/1 -> Divide3/2
  Divide3/1 -> Divide3_pd1/1
  Divide3_pd1/1 -> Out1/1

== system gm_ObjectTrackerHDL/ObjectTrackerHDL/Track/MaxCorrelation/MaxCtrl ==
  pixelIn : Inport  OutDataTypeStr=fixdt(1, 24, 16)  PortDimensions=1  SampleTime=7.94444444444444e-08
  reset : Inport  Port=2  OutDataTypeStr=boolean  PortDimensions=1  SampleTime=7.94444444444444e-08
  AND : Logic  Operator=NOT  AllPortsSameDT=off  OutDataTypeStr=boolean
  AND1 : Logic  AllPortsSameDT=off  OutDataTypeStr=boolean
  AND2 : Logic  AllPortsSameDT=off  OutDataTypeStr=boolean
  Compare To Zero : simulink/Logic and Bit Operations/Compare To Zero  relop=~=  OutDataTypeStr=boolean
  Constant3 : Constant  Value=0  OutDataTypeStr=fixdt(1,24,16)  SampleTime=-1
  Delay : Delay  DelayLength=1
  Delay4 : Delay
  Delay5 : Delay
  Delay8 : Delay  DelayLength=1
  Max : MinMax  Function=max  Inputs=2  OutDataTypeStr=fixdt(1, 24, 16)
  NOT : Logic  Operator=NOT  AllPortsSameDT=off  OutDataTypeStr=boolean
  Relational Operator : RelationalOperator  Operator=~=  OutDataTypeStr=boolean  RndMeth=Simplest  InputSameDT=off
  Relational Operator1 : RelationalOperator  Operator===  OutDataTypeStr=boolean  RndMeth=Simplest  InputSameDT=off
  Switch7 : Switch  Criteria=u2 ~= 0  OutDataTypeStr=fixdt(1, 24, 16)  SaturateOnIntegerOverflow=off  InputSameDT=off
  Switch8 : Switch  Criteria=u2 ~= 0  OutDataTypeStr=fixdt(1, 24, 16)  SaturateOnIntegerOverflow=off  InputSameDT=off
  newMaxCtrl : Outport  SampleTime=7.94444444444444e-08
  sameMaxCtrl : Outport  Port=2  SampleTime=7.94444444444444e-08
  wires:
  pixelIn/1 -> Switch7/1, Relational Operator1/1
  reset/1 -> NOT/1
  AND/1 -> AND1/1
  AND1/1 -> sameMaxCtrl/1
  AND2/1 -> Delay5/1
  Compare To Zero/1 -> AND2/2
  Constant3/1 -> Switch7/3, Switch8/3
  Delay/1 -> Relational Operator/1, Switch8/1
  Delay4/1 -> AND/1, newMaxCtrl/1
  Delay5/1 -> AND1/2
  Delay8/1 -> Switch7/2, Switch8/2
  Max/1 -> Relational Operator1/2, Relational Operator/2, Compare To Zero/1, Delay/1
  NOT/1 -> Delay8/1
  Relational Operator/1 -> Delay4/1
  Relational Operator1/1 -> AND2/1
  Switch7/1 -> Max/1
  Switch8/1 -> Max/2

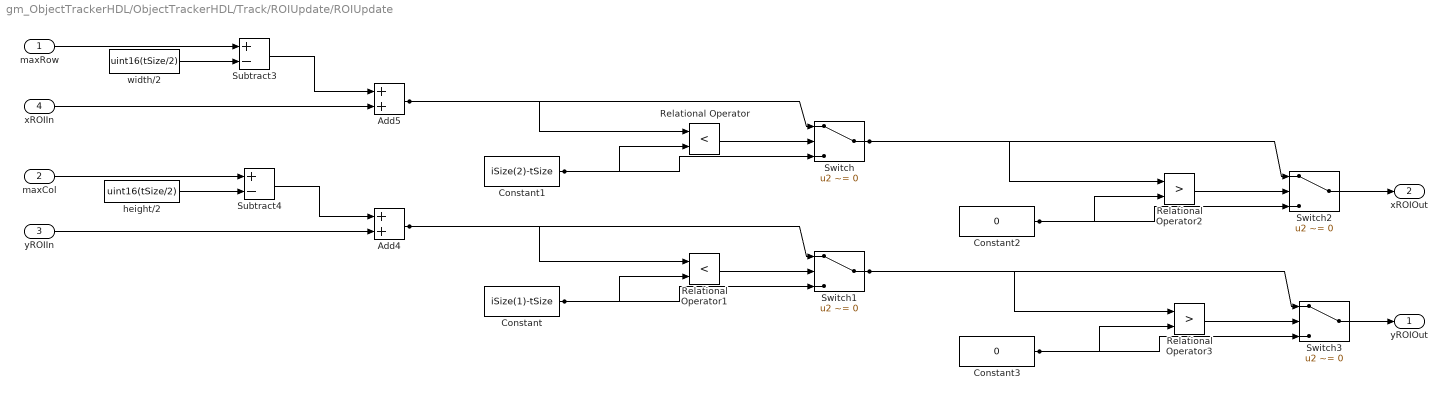
== system gm_ObjectTrackerHDL/ObjectTrackerHDL/Track/ROIUpdate/ROIUpdate ==
  maxRow : Inport  OutDataTypeStr=uint16  PortDimensions=1  SampleTime=7.94444444444444e-08
  maxCol : Inport  Port=2  OutDataTypeStr=uint16  PortDimensions=1  SampleTime=7.94444444444444e-08
  yROIIn : Inport  Port=3  OutDataTypeStr=uint16  PortDimensions=1  SampleTime=7.94444444444444e-08
  xROIIn : Inport  Port=4  OutDataTypeStr=uint16  PortDimensions=1  SampleTime=7.94444444444444e-08
  Add4 : Sum  OutDataTypeStr=fixdt(1,17,0)
  Add5 : Sum  OutDataTypeStr=fixdt(1,17,0)
  Constant : Constant  Value=iSize(1)-tSize  OutDataTypeStr=fixdt(1,17,0)  SampleTime=-1
  Constant1 : Constant  Value=iSize(2)-tSize  OutDataTypeStr=fixdt(1,17,0)  SampleTime=-1
  Constant2 : Constant  Value=0  OutDataTypeStr=fixdt(1,17,0)  SampleTime=-1
  Constant3 : Constant  Value=0  OutDataTypeStr=fixdt(1,17,0)  SampleTime=-1
  Relational Operator : RelationalOperator  Operator=<  OutDataTypeStr=boolean  RndMeth=Simplest  InputSameDT=off
  Relational Operator1 : RelationalOperator  Operator=<  OutDataTypeStr=boolean  RndMeth=Simplest  InputSameDT=off
  Relational Operator2 : RelationalOperator  Operator=>  OutDataTypeStr=boolean  RndMeth=Simplest  InputSameDT=off
  Relational Operator3 : RelationalOperator  Operator=>  OutDataTypeStr=boolean  RndMeth=Simplest  InputSameDT=off
  Subtract3 : Sum  Inputs=+-  OutDataTypeStr=fixdt(1,17,0)
  Subtract4 : Sum  Inputs=+-  OutDataTypeStr=fixdt(1,17,0)
  Switch{,1..3} (4 alike) : Switch  Criteria=u2 ~= 0  OutDataTypeStr=fixdt(1, 17, 0)  SaturateOnIntegerOverflow=off  InputSameDT=off
  height/2 : Constant  Value=uint16(tSize/2)  OutDataTypeStr=uint16  SampleTime=-1
  width/2 : Constant  Value=uint16(tSize/2)  OutDataTypeStr=uint16  SampleTime=-1
  yROIOut : Outport  SampleTime=7.94444444444444e-08
  xROIOut : Outport  Port=2  SampleTime=7.94444444444444e-08
  wires:
  maxRow/1 -> Subtract3/1
  maxCol/1 -> Subtract4/1
  yROIIn/1 -> Add4/2
  xROIIn/1 -> Add5/2
  Add4/1 -> Switch1/1, Relational Operator1/1
  Add5/1 -> Switch/1, Relational Operator/1
  Constant/1 -> Switch1/3, Relational Operator1/2
  Constant1/1 -> Switch/3, Relational Operator/2
  Constant2/1 -> Switch2/3, Relational Operator2/2
  Constant3/1 -> Switch3/3, Relational Operator3/2
  Relational Operator/1 -> Switch/2
  Relational Operator1/1 -> Switch1/2
  Relational Operator2/1 -> Switch2/2
  Relational Operator3/1 -> Switch3/2
  Subtract3/1 -> Add5/1
  Subtract4/1 -> Add4/1
  Switch/1 -> Switch2/1, Relational Operator2/1
  Switch1/1 -> Switch3/1, Relational Operator3/1
  Switch2/1 -> xROIOut/1
  Switch3/1 -> yROIOut/1
  height/2/1 -> Subtract4/2
  width/2/1 -> Subtract3/2

== system gm_ObjectTrackerHDL/ObjectTrackerHDL/Track/2-DCorrelation/2-DIFFT/CornerTurnMemory ==
  dataIn : Inport  OutDataTypeStr=fixdt(0, 64, 0)  PortDimensions=1  SampleTime=7.94444444444444e-08
  validIn : Inport  Port=2  OutDataTypeStr=boolean  PortDimensions=1  SampleTime=7.94444444444444e-08
  BankBit : Subsystem
  Bit Slice3 : hdlsllib/Logic and Bit Operations/Bit Slice  lidx=(log2(numCols)+log2(numRows))-1  ridx=0
  CounterDelay : Subsystem
  Delay : Delay  DelayLength=1
  Delay1 : Delay  DelayLength=1
  Logical Operator3 : Logic  IconShape=distinctive  AllPortsSameDT=off  OutDataTypeStr=boolean
  Logical Operator4 : Logic  IconShape=distinctive  AllPortsSameDT=off  OutDataTypeStr=boolean
  Logical Operator5 : Logic  Operator=NOT  IconShape=distinctive  AllPortsSameDT=off  OutDataTypeStr=boolean
  LowerRAM : Subsystem
  ReadAddrCntr : hdlsllib/Sources/HDL Counter  CountType=Count limited  CountInit=0  CountStep=1  CountMax=(2 * numCols * numRows) -1  CountFromType=Initial value  CountFrom=0  CountResetPort=off  CountLoadPort=off  CountEnbPort=on  CountDirPort=off  CountHitOutputPort=off  CountDataType=Unsigned  CountWordLen=log2(numCols) + log2(numRows) + 1  CountFracLen=0  CountSampTime=-1
  SwapAddr : Subsystem
  Switch1 : Switch  Criteria=u2 ~= 0  OutDataTypeStr=fixdt(0, 64, 0)  SaturateOnIntegerOverflow=off  InputSameDT=off
  UpperRAM : Subsystem
  WriteAddrCntr : hdlsllib/Sources/HDL Counter  CountType=Count limited  CountInit=0  CountStep=1  CountMax=(2 * numCols * numRows)-1  CountFromType=Initial value  CountFrom=0  CountResetPort=off  CountLoadPort=off  CountEnbPort=on  CountDirPort=off  CountHitOutputPort=off  CountDataType=Unsigned  CountWordLen=log2(numCols) + log2(numRows) + 1  CountFracLen=0  CountSampTime=-1
  dataOut : Outport  SampleTime=7.94444444444444e-08
  validOut : Outport  Port=2  SampleTime=7.94444444444444e-08
  wires:
  dataIn/1 -> UpperRAM/1(din), LowerRAM/1(din)
  validIn/1 -> Logical Operator4/2, Logical Operator3/1, CounterDelay/1(vld_in), WriteAddrCntr/1
  BankBit/1(bankWr) -> Logical Operator5/1, Logical Operator3/2
  Bit Slice3/1 -> UpperRAM/2(wr_addr), LowerRAM/2(wr_addr)
  CounterDelay/1(vld_out) -> Delay1/1, ReadAddrCntr/1
  Delay/1 -> Switch1/2
  Delay1/1 -> validOut/1
  Logical Operator3/1 -> LowerRAM/3(wr_en)
  Logical Operator4/1 -> UpperRAM/3(wr_en)
  Logical Operator5/1 -> Logical Operator4/1
  LowerRAM/1(dout) -> Switch1/1
  ReadAddrCntr/1 -> SwapAddr/1(addrIn)
  SwapAddr/1(bankRd) -> Delay/1
  SwapAddr/2(addrRd) -> UpperRAM/4(rd_addr), LowerRAM/4(rd_addr)
  Switch1/1 -> dataOut/1
  UpperRAM/1(dout) -> Switch1/3
  WriteAddrCntr/1 -> Bit Slice3/1, BankBit/1(addrIn)

== system gm_ObjectTrackerHDL/ObjectTrackerHDL/Track/2-DCorrelation/2-DIFFT/pixelBusGenerator ==
  validIn : Inport  OutDataTypeStr=boolean  PortDimensions=1  SampleTime=7.94444444444444e-08
  Horizontal : hdlsllib/Sources/HDL Counter  CountType=Count limited  CountInit=0  CountStep=1  CountMax=hEnd  CountFromType=Initial value  CountFrom=0  CountResetPort=off  CountLoadPort=off  CountEnbPort=on  CountDirPort=off  CountHitOutputPort=off  CountDataType=Unsigned  CountWordLen=ceil(log2(hEnd))  CountFracLen=0  CountSampTime=1
  Logical Operator{3..6} (4 alike) : Logic  AllPortsSameDT=off  OutDataTypeStr=boolean
  Pixel Control Bus Creator : Subsystem  mask(Pixel Control Bus Creator){}
      mask help:
      | Creates a pixelcontrol bus. The block has 5 input ports:
      |
      | hStart - First pixel in a horizontal line of a frame
      | hEnd - Last pixel in a horizontal line of a frame
      | vStart - First pixel in the first (top) line of a frame
      | vEnd - Last pixel in the last (bottom) line of a frame
      | valid - Valid pixel indicator
      mask Display:
      | disp('Pixel Control\nBus Creator');
      | port_label('input',1,'hStart');
      | port_label('input',2,'hEnd');
      | port_label('input',3,'vStart');
      | port_label('input',4,'vEnd');
      | port_label('input',5,'valid');
      | port_label('output',1,'ctrl');
  Vertical : hdlsllib/Sources/HDL Counter  CountType=Count limited  CountInit=0  CountStep=1  CountMax=vEnd  CountFromType=Initial value  CountFrom=0  CountResetPort=off  CountLoadPort=off  CountEnbPort=on  CountDirPort=off  CountHitOutputPort=off  CountDataType=Unsigned  CountWordLen=ceil(log2(vEnd))  CountFracLen=0  CountSampTime=1
  hEnd : simulink/Logic and Bit Operations/Compare To Constant  relop===  const=hEnd  OutDataTypeStr=boolean
  hStart : simulink/Logic and Bit Operations/Compare To Constant  relop===  const=0  OutDataTypeStr=boolean
  vEnd : simulink/Logic and Bit Operations/Compare To Constant  relop===  const=vEnd  OutDataTypeStr=boolean
  vStart : simulink/Logic and Bit Operations/Compare To Constant  relop===  const=0  OutDataTypeStr=boolean
  busOut : Outport  VectorParamsAs1DForOutWhenUnconnected=off
  wires:
  validIn/1 -> Logical Operator6/1, Logical Operator5/1, Logical Operator4/1, Logical Operator3/1, Pixel Control Bus Creator/5(In5), Vertical/1, Horizontal/1
  Horizontal/1 -> hStart/1, hEnd/1
  Logical Operator3/1 -> Pixel Control Bus Creator/1(In1)
  Logical Operator4/1 -> Pixel Control Bus Creator/2(In2)
  Logical Operator5/1 -> Pixel Control Bus Creator/3(In3)
  Logical Operator6/1 -> Pixel Control Bus Creator/4(In4)
  Pixel Control Bus Creator/1(Out1) -> busOut/1
  Vertical/1 -> vStart/1, vEnd/1
  hEnd/1 -> Logical Operator4/2
  hStart/1 -> Logical Operator3/2
  vEnd/1 -> Logical Operator6/2
  vStart/1 -> Logical Operator5/2

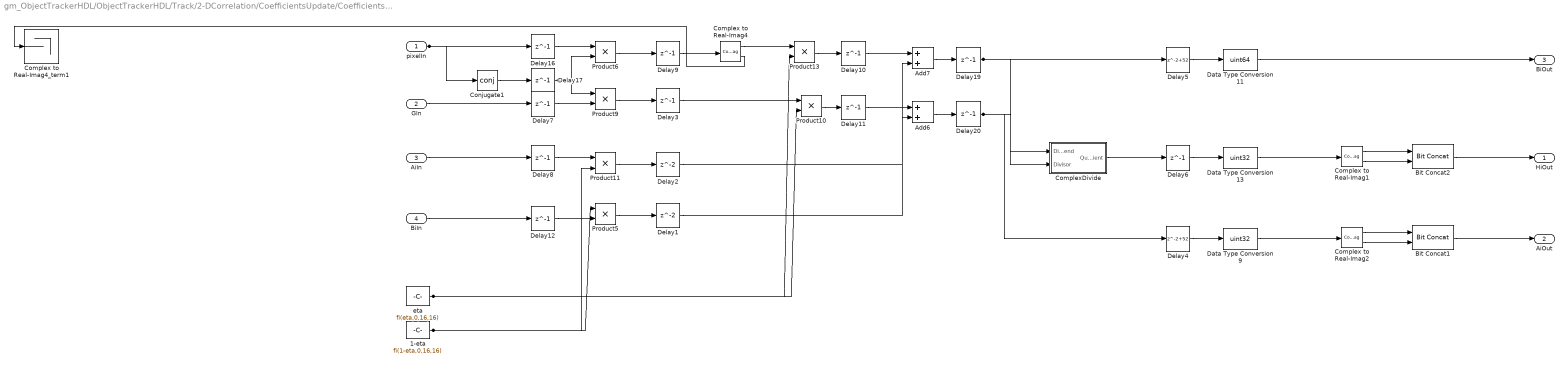
== system gm_ObjectTrackerHDL/ObjectTrackerHDL/Track/2-DCorrelation/CoefficientsUpdate/CoefficientsUpdate ==
  pixelIn : Inport  OutDataTypeStr=fixdt(1, 24, 12)  PortDimensions=1  SampleTime=7.94444444444444e-08
      settings: SignalType=complex
  GIn : Inport  Port=2  OutDataTypeStr=fixdt(1, 16, 11)  PortDimensions=1  SampleTime=7.94444444444444e-08
  AiIn : Inport  Port=3  OutDataTypeStr=fixdt(1, 28, 8)  PortDimensions=1  SampleTime=7.94444444444444e-08
      settings: SignalType=complex
  BiIn : Inport  Port=4  OutDataTypeStr=fixdt(1, 36, 8)  PortDimensions=1  SampleTime=7.94444444444444e-08
  1-eta : Constant  Value=fi(1-eta,0,16,16)  OutDataTypeStr=fixdt(0,16,16)  SampleTime=-1
  Add6 : Sum  OutDataTypeStr=fixdt(1,28,8)
  Add7 : Sum  OutDataTypeStr=fixdt(1,36,8)
  Bit Concat1 : hdlsllib/Logic and Bit Operations/Bit Concat  numInputs=2
  Bit Concat2 : hdlsllib/Logic and Bit Operations/Bit Concat  numInputs=2
  Complex to Real-Imag1 : ComplexToRealImag
  Complex to Real-Imag2 : ComplexToRealImag
  Complex to Real-Imag4 : ComplexToRealImag
  Complex to Real-Imag4_term1 : Terminator
  ComplexDivide : Subsystem
  Conjugate1 : Math  Operator=conj  SignedPower=on  OutDataTypeStr=fixdt(1, 24, 12)  RndMeth=Zero
  Data Type Conversion11 : DataTypeConversion  OutDataTypeStr=uint64  ConvertRealWorld=Stored Integer (SI)  SaturateOnIntegerOverflow=off  RndMeth=Floor
  Data Type Conversion13 : DataTypeConversion  OutDataTypeStr=uint32  ConvertRealWorld=Stored Integer (SI)  SaturateOnIntegerOverflow=off  RndMeth=Floor
  Data Type Conversion9 : DataTypeConversion  OutDataTypeStr=uint32  ConvertRealWorld=Stored Integer (SI)  SaturateOnIntegerOverflow=off  RndMeth=Floor
  Delay1 : Delay  InitialCondition=0
  Delay{3,6..12,16..17,19..20} (12 alike) : Delay  DelayLength=1  InitialCondition=0
  Delay2 : Delay  InitialCondition=0
  Delay4 : Delay  DelayLength=2+52  InitialCondition=0
  Delay5 : Delay  DelayLength=2+52  InitialCondition=0
  Product10 : Product  OutDataTypeStr=fixdt(1,24,12)
  Product11 : Product  OutDataTypeStr=fixdt(1,28,8)
  Product13 : Product  OutDataTypeStr=fixdt(1,32,12)
  Product5 : Product  OutDataTypeStr=fixdt(1,36,8)
  Product6 : Product  OutDataTypeStr=fixdt(1,32,8)
  Product9 : Product  OutDataTypeStr=fixdt(1,24,8)
  eta : Constant  Value=fi(eta,0,16,16)  OutDataTypeStr=fixdt(0, 16, 16)  SampleTime=-1
  HiOut : Outport  SampleTime=7.94444444444444e-08
  AiOut : Outport  Port=2  SampleTime=7.94444444444444e-08
  BiOut : Outport  Port=3  SampleTime=7.94444444444444e-08
  wires:
  pixelIn/1 -> Delay16/1, Conjugate1/1
  GIn/1 -> Delay7/1
  AiIn/1 -> Delay8/1
  BiIn/1 -> Delay12/1
  1-eta/1 -> Product5/1, Product11/2
  Add6/1 -> Delay20/1
  Add7/1 -> Delay19/1
  Bit Concat1/1 -> AiOut/1
  Bit Concat2/1 -> HiOut/1
  Complex to Real-Imag1/1 -> Bit Concat2/1
  Complex to Real-Imag1/2 -> Bit Concat2/2
  Complex to Real-Imag2/1 -> Bit Concat1/1
  Complex to Real-Imag2/2 -> Bit Concat1/2
  Complex to Real-Imag4/1 -> Product13/1
  Complex to Real-Imag4/2 -> Complex to Real-Imag4_term1/1
  ComplexDivide/1(Quotient) -> Delay6/1
  Conjugate1/1 -> Delay17/1
  Data Type Conversion11/1 -> BiOut/1
  Data Type Conversion13/1 -> Complex to Real-Imag1/1
  Data Type Conversion9/1 -> Complex to Real-Imag2/1
  Delay1/1 -> Add7/2
  Delay10/1 -> Add7/1
  Delay11/1 -> Add6/1
  Delay12/1 -> Product5/2
  Delay16/1 -> Product6/1
  Delay17/1 -> Product9/1, Product6/2
  Delay19/1 -> Delay5/1, ComplexDivide/2(Divisor)
  Delay2/1 -> Add6/2
  Delay20/1 -> Delay4/1, ComplexDivide/1(Dividend)
  Delay3/1 -> Product10/1
  Delay4/1 -> Data Type Conversion9/1
  Delay5/1 -> Data Type Conversion11/1
  Delay6/1 -> Data Type Conversion13/1
  Delay7/1 -> Product9/2
  Delay8/1 -> Product11/1
  Delay9/1 -> Complex to Real-Imag4/1
  Product10/1 -> Delay11/1
  Product11/1 -> Delay2/1
  Product13/1 -> Delay10/1
  Product5/1 -> Delay1/1
  Product6/1 -> Delay9/1
  Product9/1 -> Delay3/1
  eta/1 -> Product13/2, Product10/2
